simulink model "ac7_example2"  (Simulink 7.8)
settings: Solver=FixedStepDiscrete  StartTime=0.0  StopTime=2  RelTol=1e-3
PreLoadFcn:
  | Ts=2e-6;
libraries: powerlib x3, AC7DriveInternalModels x2, powerlib_extras x2, electricdrivelib x1
Description:
  | Copyright 2008-2011 The MathWorks, Inc.
settings Model: Creator=MathWorks  LastModifiedBy=Harvey  ExtModeAutoUpdateStatusClock=off
settings DataIOCC: SignalLoggingName=sigsOut
settings OptimizationCC: InlineInvariantSignals=on  InitFltsAndDblsToZero=on
settings DebuggingCC: CheckExecutionContextPreStartOutputMsg=on  CheckExecutionContextRuntimeOutputMsg=on  SignalResolutionControl=TryResolveAllWithWarning  SolverPrmCheckMsg=none  MultiTaskDSMMsg=warning  MultiTaskCondExecSysMsg=none  FcnCallInpInsideContextMsg=Use local settings  UnconnectedLineMsg=none  StrictBusMsg=None
settings HardwareCC: TargetUnknown=on
settings RTWCC: IncludeERTFirstTime=on

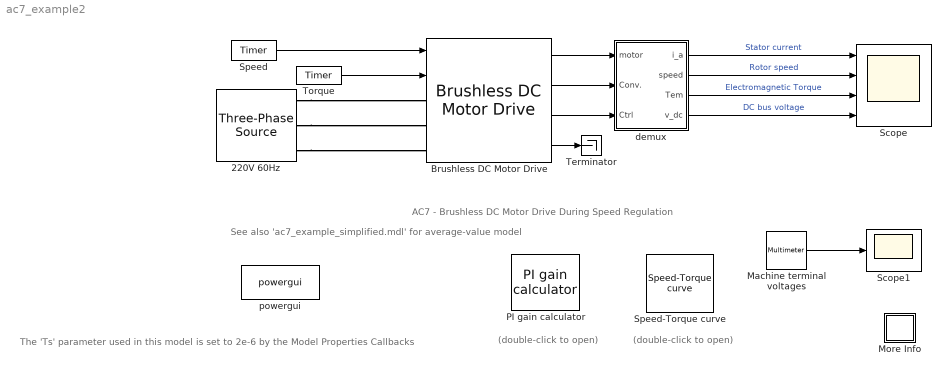
== system ac7_example2 ==
  note: AC7 - Brushless DC Motor Drive During Speed Regulation
  note: The 'Ts' parameter used in this model
      | is set to 2e-6  by the Model Properties Callbacks
  note: See also 'ac7_example_simplified.mdl' for average-value model
  note: (double-click to open)
  note: (double-click to open)
  220V 60Hz : powerlib/Electrical Sources/Three-Phase Source  Voltage=220  PhaseAngle=0  Frequency=60  InternalConnection=Yg  SpecifyImpedance=off  Resistance=0.02  Inductance=0.05e-3  ShortCircuitLevel=100e6  BaseVoltage=25e3  XRratio=7  BusType=swing  Pref=0  Qref=0  Qmin=-inf  Qmax=inf
  Brushless DC Motor Drive : electricdrivelib/AC drives/Brushless DC Motor Drive  showMaskWarnings=on  AverageValue=off  MechanicalLoad=Torque Tm  driveType=AC7
  Machine terminal voltages : powerlib/Measurements/Multimeter  PhasorSimulation=off  OutputType=Complex  sel=1  L=32  Gain=0  yselected={}  PSBOutputType=1  PSBequivalent=0  AxesSetting=[0,0.1,-100,100]  Display=0  SavedBlockNames=-11
  More Info : Subsystem
      settings: OpenFcn=showdemo(bdroot(gcb))
      mask Display: disp('?')
  PI gain calculator : AC7DriveInternalModels/PI gain calculator  mec=[0.089 0.005 4]  specs=on  ele=[0.2 8.5e-3]  lam=0.175  open_loop=off  zeta=0.99  Trd=0.13/5  check=off
  Scope : Scope  NumInputPorts=4
      settings: TimeRange=2  YMin=-15~300~-20~305.5  YMax=10~440~12.5~307.75  SaveName=simout  Decimation=25
  Scope1 : Scope
  Speed : powerlib_extras/Control  Blocks/Timer  t=[0 1 ]  e=[300 0]
  Speed-Torque curve : AC7DriveInternalModels/Speed-Torque curve  ele=[0.2 8.5e-3]  Flux=0.175  mec=[0.089 0.005 4]  Vdc=310  Tmax=17.8  accel=1000  check=off
  Terminator : Terminator
  Torque : powerlib_extras/Control  Blocks/Timer  t=[0.5 1.5]  e=[11 -11]
  demux : Subsystem
  powergui : powerlib/powergui  SimulationMode=Discrete  SolverType=Tustin  SampleTime=Ts  frequency=60  SPID=off  DisableSnubberDevices=off  DisableRonSwitches=off  DisableVfSwitches=off  SwTol=0  Interpol=off  DisplayEquations=off  FunctionMessages=off  frequencyindice=60  Pbase=100e6  ErrMax=1e-4  Iterations=50  UnitsV=kV  UnitsW=MW  echomessages=off  HookPort=off  EnableUseOfTLC=off  x0status=blocks  RestoreLinks=warning  ResistiveCurrentMeasurement=off  Frange=[0:2:500]  Ylog=off  Xlog=on  ShowGrid=off  save=off  variable=ZData  ZoomFFT=on  StartTime=0.0  cycles=1  DisplayStyle=1  fundamental=60  FreqAxis=off  MaxFrequency=1000  frequencyindicesteady=1  RmsSteady=1  display=off  Ts=0  methode=off
  wires:
  Brushless DC Motor Drive/1 -> demux/1(motor)
  Brushless DC Motor Drive/2 -> demux/2(Conv.)
  Brushless DC Motor Drive/3 -> demux/3(Ctrl)
  demux/1(i_a) -> Scope/1  "Stator current"
  demux/2(speed) -> Scope/2  "Rotor speed"
  demux/3(Tem) -> Scope/3  "Electromagnetic Torque"
  demux/4(v_dc) -> Scope/4  "DC bus voltage"
  Machine terminal voltages/1 -> Scope1/1
  Speed/1 -> Brushless DC Motor Drive/1
  Torque/1 -> Brushless DC Motor Drive/2
  Brushless DC Motor Drive/4 -> Terminator/1
  connections:
  220V 60Hz/RConn1 -- Brushless DC Motor Drive/LConn1
  220V 60Hz/RConn2 -- Brushless DC Motor Drive/LConn2
  220V 60Hz/RConn3 -- Brushless DC Motor Drive/LConn3

== system ac7_example2/More Info ==

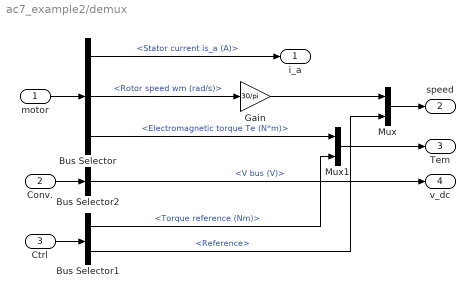
== system ac7_example2/demux ==
  motor : Inport
  Conv. : Inport  Port=2
  Ctrl : Inport  Port=3
  Bus Selector : BusSelector  OutputSignals=Stator current is_a (A),Rotor speed wm (rad/s),Electromagnetic torque Te (N*m)
  Bus Selector1 : BusSelector  OutputSignals=Torque reference (Nm),Reference
  Bus Selector2 : BusSelector  OutputSignals=V bus (V)
  Gain : Gain  Gain=30/pi  SaturateOnIntegerOverflow=on  OutDataTypeStr=Inherit: Same as input  ParamDataTypeStr=Inherit: Same as input
  Mux : Mux  Inputs=2
  Mux1 : Mux  Inputs=2
  i_a : Outport
  speed : Outport  Port=2
  Tem : Outport  Port=3
  v_dc : Outport  Port=4
  wires:
  Bus Selector/2 -> Gain/1  "<Rotor speed wm (rad/s)>"
  Bus Selector2/1 -> v_dc/1  "<V bus (V)>"
  Conv./1 -> Bus Selector2/1
  Ctrl/1 -> Bus Selector1/1
  Bus Selector1/1 -> Mux1/2  "<Torque reference (Nm)>"
  Bus Selector1/2 -> Mux/2  "<Reference>"
  Gain/1 -> Mux/1
  Bus Selector/1 -> i_a/1  "<Stator current is_a (A)>"
  Bus Selector/3 -> Mux1/1  "<Electromagnetic torque Te (N*m)>"
  Mux1/1 -> Tem/1
  Mux/1 -> speed/1
  motor/1 -> Bus Selector/1
